simulink model "cubesat_alg_dev_env_v2_main"  (R2023a)
settings: Solver=FixedStepAuto  StartTime=0.0  StopTime=7200  FixedStep=0.01  MaxStep=1  MinStep=0.01  RelTol=1e-3
model workspace (MAT data in the model file):
  visSampleTime = 3
undefined symbols (not defined in the file or in its folder): WMM2020
libraries: aerolibutil x9, matrix_library x6, vrlib x4, sharedtransform x2, aerolibgravity2 x2, dspinverses x1, sharedutil x1, simulink_extras x1
(part 2 of 2)

== matlab function cubesat_alg_dev_env_v2_main/env_modelling/MATLAB Function ==
  data: pos_gci input; torque_body output; iner_tensor input
function torque_body  = grav_grad_torque(pos_gci, iner_tensor)
    % mass of earth, grav constant
    m_e = 5.97219e24;
    G = 6.67430e-11;

    % grav param
    u = G*m_e;

    radius = norm(pos_gci);
    nadir_vec = -normalize(pos_gci);
    torque_body = cross(3*u/radius^3*nadir_vec, ...
        iner_tensor*nadir_vec);

== matlab function cubesat_alg_dev_env_v2_main/datetime_modelling_and_ref_frames/MATLAB Function1 ==
  data: datetime input; dyear output
function dyear = dyear_from_datetime(datetime)

    % the datetime format is provided as a 6 value array
    % year, month, day, hour, minute, second

    % sequentially builds the decimal year

    % potentially we may want to use /61 for leap second days but this is
    % likely fine as our simulation just needs to perform regular datetime
    % updates for simple testing

    tot_mins = datetime(5) + datetime(6) / 60;
    tot_hours = datetime(4) + tot_mins / 60;
    tot_days = datetime(3) + tot_hours / 24;
    tot_months = datetime(2) + tot_days / (275/9); % average days in month across year
    tot_years = datetime(1) + tot_months / 12;

    dyear = tot_years;

== matlab function cubesat_alg_dev_env_v2_main/onboad_env_modelling/MATLAB Function6 ==
  data: u input; y output
function y = noise_sim(u)

y = u;

== matlab function cubesat_alg_dev_env_v2_main/sens_modelling/MATLAB Function2 ==
  data: in input; out output; max_value input; min_value input
function out = zero_out_out_of_range(in, max_value, min_value)
    out = in;

    for i = 1:length(in)
        if out(i) < min_value || out(i) > max_value
            out(i) = 0;
        end
    end
